simulink model "SecRwLtStArmScrnIsPosChk"  (R2018b)
settings: Solver=FixedStepDiscrete  StartTime=0.0  StopTime=10.0  FixedStep=0.01  RelTol=1e-3
undefined symbols (not defined in the file or in its folder): KeSMSuSecRwStArmTochPosDelta_Val, KeSMSuSecRwStArmTochPosTolr_Val
libraries: simulink x5, StIsPosChkLib x4
settings Model: Creator=sn2xws  LastModifiedBy=sn2xws
settings DataIOCC: SaveFormat=StructureWithTime
settings OptimizationCC: DefaultParameterBehavior=Inlined  EnhancedBackFolding=on  PassReuseOutputArgsAs=Individual arguments  ZeroExternalMemoryAtStartup=off  ZeroInternalMemoryAtStartup=off  OptimizeBlockOrder=speed  DifferentSizesBufferReuse=on  OptimizationCustomize=off
settings DebuggingCC: ParameterTunabilityLossMsg=error
settings ModelReferenceCC: ModelReferenceNumInstancesAllowed=Single
settings SFSimCC: MATLABDynamicMemAlloc=off
settings RTWCC: SystemTargetFile=autosar.tlc  GenCodeOnly=on  TemplateMakefile=ert_default_tmf  Description=AUTOSAR  GenerateReport=on  IncludeHyperlinkInReport=on  LaunchReport=on  GenerateTraceInfo=on  GenerateTraceReport=on  GenerateTraceReportSl=on  GenerateTraceReportSf=on  GenerateTraceReportEml=on  GenerateCodeMetricsReport=on
settings CodeAppCC: ForceParamTrailComments=on  IgnoreCustomStorageClasses=off  OperatorAnnotations=on  SimulinkDataObjDesc=on  SFDataObjDesc=on  InsertBlockDesc=on
settings STFCustomTargetCC: TargetLangStandard=C99 (ISO)  MultiwordLength=256  ParMdlRefBuildCompliant=on  CompOptLevelCompliant=on  IncludeMdlTerminateFcn=off  CombineOutputUpdateFcns=on  SuppressErrorStatus=on  ERTCustomFileBanners=on  SupportNonFinite=off  SupportComplex=off  SupportContinuousTime=off  SupportNonInlinedSFcns=off  RemoveResetFunc=on  MATLABClassNameForMDSCustomization=Simulink.SoftwareTarget.ERTCustomization  AutosarCompliant=on  UseToolchainInfoCompliant=on  LookupTableObjectStructAxisOrder=2,1,3,4,...  LUTObjectStructOrderEvenSpacing=Size,Table,Breakpoints  SystemTargetFile=autosar.tlc
settings ERTTargetCC: TargetLangStandard=C99 (ISO)  ConcurrentExecutionCompliant=off  IncludeMdlTerminateFcn=off  SuppressErrorStatus=on  SupportNonFinite=off  SupportComplex=off  ModelStepFunctionPrototypeControlCompliant=off  CPPClassGenCompliant=off  AutosarCompliant=on  LookupTableObjectStructAxisOrder=2,1,3,4,...  LUTObjectStructOrderEvenSpacing=Size,Table,Breakpoints  InlinedParameterPlacement=NonHierarchical  ERTCustomFileTemplate=example_file_process.tlc  ERTFilePackagingFormat=Compact

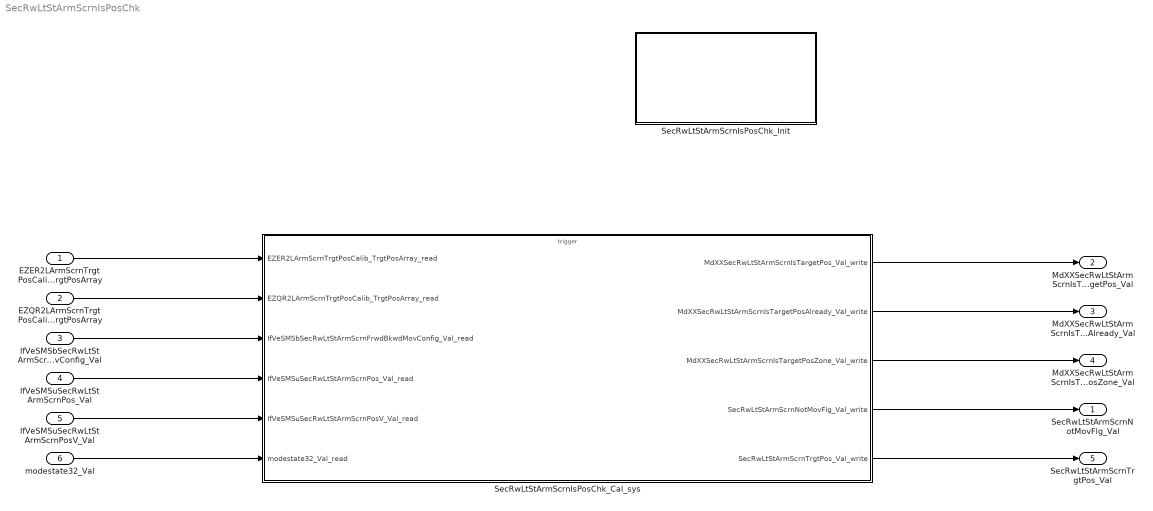
== system SecRwLtStArmScrnIsPosChk ==
  EZER2LArmScrnTrgtPosCalib_TrgtPosArray : Inport  Description=|  OutDataTypeStr=uint16  PortDimensions=3
      | 0:Pos
      | 1:Max
      | 2:Min
  EZQR2LArmScrnTrgtPosCalib_TrgtPosArray : Inport  Description=|  Port=2  OutDataTypeStr=uint16  PortDimensions=3
      | 0:Pos
      | 1:Max
      | 2:Min
  IfVeSMSbSecRwLtStArmScrnFrwdBkwdMovConfig_Val : Inport  Port=3  OutDataTypeStr=boolean  PortDimensions=1
  IfVeSMSuSecRwLtStArmScrnPos_Val : Inport  Port=4  OutDataTypeStr=uint16  PortDimensions=1
  IfVeSMSuSecRwLtStArmScrnPosV_Val : Inport  Port=5  OutDataTypeStr=boolean  PortDimensions=1
  modestate32_Val : Inport  Port=6  OutDataTypeStr=uint32  PortDimensions=1
  SecRwLtStArmScrnIsPosChk_Cal_sys : Subsystem
  SecRwLtStArmScrnIsPosChk_Init : Subsystem
  SecRwLtStArmScrnNotMovFlg_Val : Outport  OutDataTypeStr=boolean  PortDimensions=1
  MdXXSecRwLtStArmScrnIsTargetPos_Val : Outport  Port=2  OutDataTypeStr=uint32  PortDimensions=1
  MdXXSecRwLtStArmScrnIsTargetPosAlready_Val : Outport  Port=3  OutDataTypeStr=uint32  PortDimensions=1
  MdXXSecRwLtStArmScrnIsTargetPosZone_Val : Outport  Port=4  OutDataTypeStr=uint32  PortDimensions=1
  SecRwLtStArmScrnTrgtPos_Val : Outport  Port=5  OutDataTypeStr=uint16  PortDimensions=1
  wires:
  EZER2LArmScrnTrgtPosCalib_TrgtPosArray/1 -> SecRwLtStArmScrnIsPosChk_Cal_sys/1(EZER2LArmScrnTrgtPosCalib_TrgtPosArray_read)
  EZQR2LArmScrnTrgtPosCalib_TrgtPosArray/1 -> SecRwLtStArmScrnIsPosChk_Cal_sys/2(EZQR2LArmScrnTrgtPosCalib_TrgtPosArray_read)
  IfVeSMSbSecRwLtStArmScrnFrwdBkwdMovConfig_Val/1 -> SecRwLtStArmScrnIsPosChk_Cal_sys/3(IfVeSMSbSecRwLtStArmScrnFrwdBkwdMovConfig_Val_read)
  IfVeSMSuSecRwLtStArmScrnPos_Val/1 -> SecRwLtStArmScrnIsPosChk_Cal_sys/4(IfVeSMSuSecRwLtStArmScrnPos_Val_read)
  IfVeSMSuSecRwLtStArmScrnPosV_Val/1 -> SecRwLtStArmScrnIsPosChk_Cal_sys/5(IfVeSMSuSecRwLtStArmScrnPosV_Val_read)
  modestate32_Val/1 -> SecRwLtStArmScrnIsPosChk_Cal_sys/6(modestate32_Val_read)
  SecRwLtStArmScrnIsPosChk_Cal_sys/5(SecRwLtStArmScrnTrgtPos_Val_write) -> SecRwLtStArmScrnTrgtPos_Val/1
  SecRwLtStArmScrnIsPosChk_Cal_sys/1(MdXXSecRwLtStArmScrnIsTargetPos_Val_write) -> MdXXSecRwLtStArmScrnIsTargetPos_Val/1
  SecRwLtStArmScrnIsPosChk_Cal_sys/2(MdXXSecRwLtStArmScrnIsTargetPosAlready_Val_write) -> MdXXSecRwLtStArmScrnIsTargetPosAlready_Val/1
  SecRwLtStArmScrnIsPosChk_Cal_sys/3(MdXXSecRwLtStArmScrnIsTargetPosZone_Val_write) -> MdXXSecRwLtStArmScrnIsTargetPosZone_Val/1
  SecRwLtStArmScrnIsPosChk_Cal_sys/4(SecRwLtStArmScrnNotMovFlg_Val_write) -> SecRwLtStArmScrnNotMovFlg_Val/1

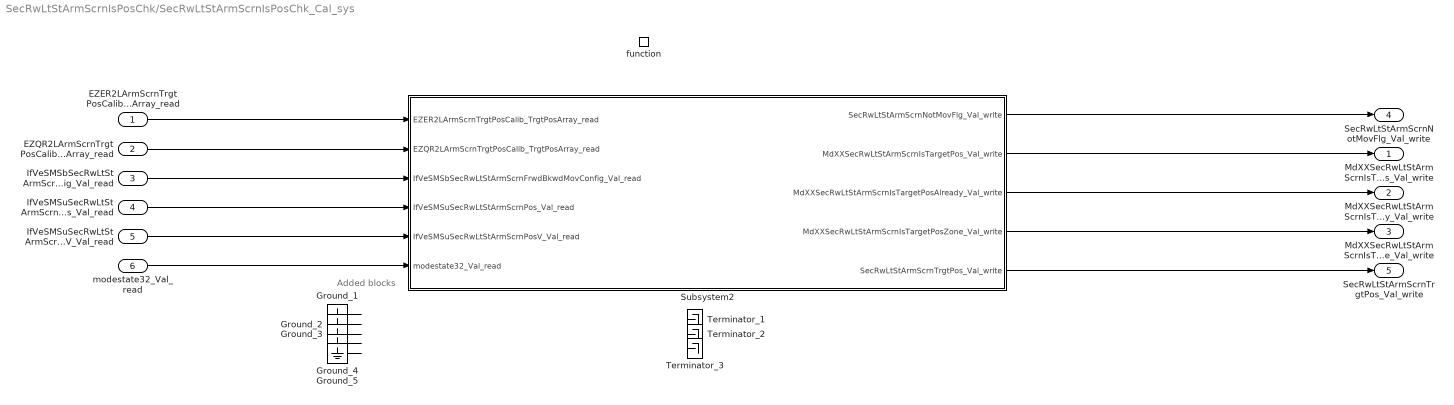
== system SecRwLtStArmScrnIsPosChk/SecRwLtStArmScrnIsPosChk_Cal_sys ==
  note: Added blocks
  EZER2LArmScrnTrgtPosCalib_TrgtPosArray_read : Inport
  EZQR2LArmScrnTrgtPosCalib_TrgtPosArray_read : Inport  Port=2
  IfVeSMSbSecRwLtStArmScrnFrwdBkwdMovConfig_Val_read : Inport  Port=3
  IfVeSMSuSecRwLtStArmScrnPos_Val_read : Inport  Port=4
  IfVeSMSuSecRwLtStArmScrnPosV_Val_read : Inport  Port=5
  modestate32_Val_read : Inport  Port=6
  function : TriggerPort  TriggerType=function-call  IsSimulinkFunction=on  FunctionName=SecRwLtStArmScrnIsPosChk_Cal  VariantControl=(inherit)
  Ground_{1..5} (5 alike) : Ground
  Subsystem2 : Subsystem
  Terminator_1 : Terminator
  Terminator_2 : Terminator
  Terminator_3 : Terminator
  MdXXSecRwLtStArmScrnIsTargetPos_Val_write : Outport
      settings: EnsureOutportIsVirtual=on
  MdXXSecRwLtStArmScrnIsTargetPosAlready_Val_write : Outport  Port=2
      settings: EnsureOutportIsVirtual=on
  MdXXSecRwLtStArmScrnIsTargetPosZone_Val_write : Outport  Port=3
      settings: EnsureOutportIsVirtual=on
  SecRwLtStArmScrnNotMovFlg_Val_write : Outport  Port=4
      settings: EnsureOutportIsVirtual=on
  SecRwLtStArmScrnTrgtPos_Val_write : Outport  Port=5
      settings: EnsureOutportIsVirtual=on
  wires:
  EZER2LArmScrnTrgtPosCalib_TrgtPosArray_read/1 -> Subsystem2/1(EZER2LArmScrnTrgtPosCalib_TrgtPosArray_read)
  EZQR2LArmScrnTrgtPosCalib_TrgtPosArray_read/1 -> Subsystem2/2(EZQR2LArmScrnTrgtPosCalib_TrgtPosArray_read)
  IfVeSMSbSecRwLtStArmScrnFrwdBkwdMovConfig_Val_read/1 -> Subsystem2/3(IfVeSMSbSecRwLtStArmScrnFrwdBkwdMovConfig_Val_read)
  IfVeSMSuSecRwLtStArmScrnPos_Val_read/1 -> Subsystem2/4(IfVeSMSuSecRwLtStArmScrnPos_Val_read)
  IfVeSMSuSecRwLtStArmScrnPosV_Val_read/1 -> Subsystem2/5(IfVeSMSuSecRwLtStArmScrnPosV_Val_read)
  modestate32_Val_read/1 -> Subsystem2/6(modestate32_Val_read)
  Subsystem2/1(SecRwLtStArmScrnNotMovFlg_Val_write) -> SecRwLtStArmScrnNotMovFlg_Val_write/1
  Subsystem2/2(MdXXSecRwLtStArmScrnIsTargetPos_Val_write) -> MdXXSecRwLtStArmScrnIsTargetPos_Val_write/1
  Subsystem2/3(MdXXSecRwLtStArmScrnIsTargetPosAlready_Val_write) -> MdXXSecRwLtStArmScrnIsTargetPosAlready_Val_write/1
  Subsystem2/4(MdXXSecRwLtStArmScrnIsTargetPosZone_Val_write) -> MdXXSecRwLtStArmScrnIsTargetPosZone_Val_write/1
  Subsystem2/5(SecRwLtStArmScrnTrgtPos_Val_write) -> SecRwLtStArmScrnTrgtPos_Val_write/1
  Ground_1/1 -> ?
  Ground_2/1 -> ?
  Ground_3/1 -> ?
  Ground_4/1 -> ?
  Ground_5/1 -> ?
  ? -> Terminator_1/1
  ? -> Terminator_2/1
  ? -> Terminator_3/1

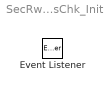
== system SecRwLtStArmScrnIsPosChk/SecRwLtStArmScrnIsPosChk_Init ==
  Event Listener : EventListener  EventName=reset

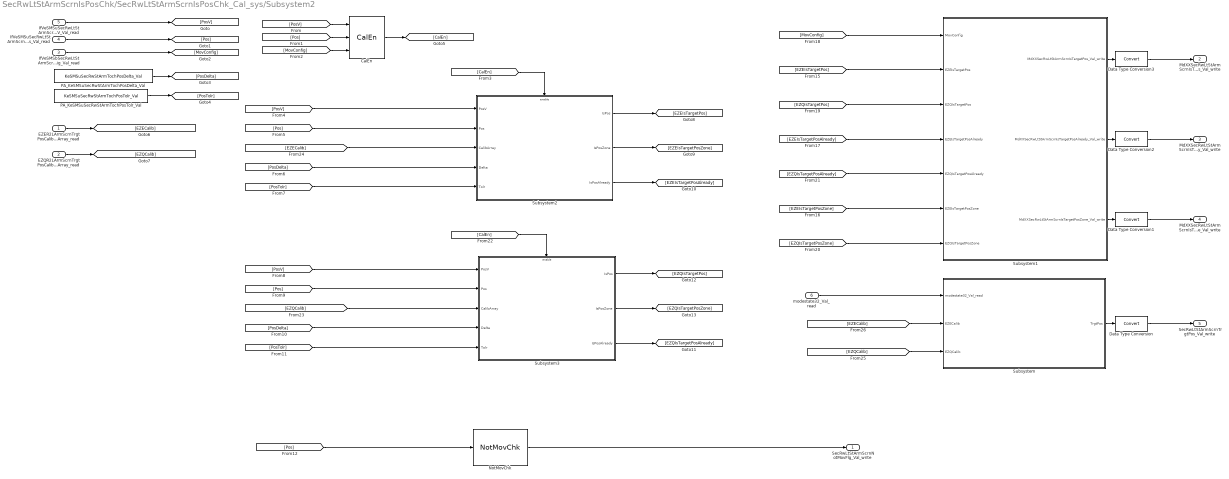
== system SecRwLtStArmScrnIsPosChk/SecRwLtStArmScrnIsPosChk_Cal_sys/Subsystem2 ==
  EZER2LArmScrnTrgtPosCalib_TrgtPosArray_read : Inport
  EZQR2LArmScrnTrgtPosCalib_TrgtPosArray_read : Inport  Port=2
  IfVeSMSbSecRwLtStArmScrnFrwdBkwdMovConfig_Val_read : Inport  Port=3
  IfVeSMSuSecRwLtStArmScrnPos_Val_read : Inport  Port=4
  IfVeSMSuSecRwLtStArmScrnPosV_Val_read : Inport  Port=5
  modestate32_Val_read : Inport  Port=6
  CalEn : StIsPosChkLib/CalEn  SystemSampleTime=-1
  Data Type Conversion{,1..3} (4 alike) : DataTypeConversion
  NotMovChk : StIsPosChkLib/NotMovChk  SystemSampleTime=-1
  PA_KeSMSuSecRwStArmTochPosDelta_Val : Constant  Value=KeSMSuSecRwStArmTochPosDelta_Val
  PA_KeSMSuSecRwStArmTochPosTolr_Val : Constant  Value=KeSMSuSecRwStArmTochPosTolr_Val
  Subsystem : Subsystem
  Subsystem1 : Subsystem
  Subsystem2 : Subsystem
  Subsystem3 : Subsystem
  SecRwLtStArmScrnNotMovFlg_Val_write : Outport
      settings: EnsureOutportIsVirtual=on
  MdXXSecRwLtStArmScrnIsTargetPos_Val_write : Outport  Port=2
      settings: EnsureOutportIsVirtual=on
  MdXXSecRwLtStArmScrnIsTargetPosAlready_Val_write : Outport  Port=3
      settings: EnsureOutportIsVirtual=on
  MdXXSecRwLtStArmScrnIsTargetPosZone_Val_write : Outport  Port=4
      settings: EnsureOutportIsVirtual=on
  SecRwLtStArmScrnTrgtPos_Val_write : Outport  Port=5
      settings: EnsureOutportIsVirtual=on
  wires:
  [PosV] -> Subsystem2/1(PosV)
  EZQR2LArmScrnTrgtPosCalib_TrgtPosArray_read/1 -> [EZQCalib]
  PA_KeSMSuSecRwStArmTochPosDelta_Val/1 -> [PosDelta]
  [MovConfig] -> Subsystem1/1(MovConfig)
  IfVeSMSuSecRwLtStArmScrnPosV_Val_read/1 -> [PosV]
  Subsystem3/1(IsPos) -> [EZQIsTargetPos]
  Data Type Conversion2/1 -> MdXXSecRwLtStArmScrnIsTargetPosAlready_Val_write/1
  NotMovChk/1 -> SecRwLtStArmScrnNotMovFlg_Val_write/1
  Data Type Conversion3/1 -> MdXXSecRwLtStArmScrnIsTargetPos_Val_write/1
  PA_KeSMSuSecRwStArmTochPosTolr_Val/1 -> [PosTolr]
  [EZEIsTargetPos] -> Subsystem1/2(EZEIsTargetPos)
  [PosDelta] -> Subsystem2/4(Delta)
  [PosDelta] -> Subsystem3/4(Delta)
  [PosTolr] -> Subsystem2/5(Tolr)
  [Pos] -> Subsystem2/2(Pos)
  Data Type Conversion/1 -> SecRwLtStArmScrnTrgtPos_Val_write/1
  Subsystem1/2(MdXXSecRwLtStArmScrnIsTargetPosAlready_Val_write) -> Data Type Conversion2/1
  [EZQIsTargetPos] -> Subsystem1/3(EZQIsTargetPos)
  Subsystem3/3(IsPosAlready) -> [EZQIsTargetPosAlready]
  Subsystem1/1(MdXXSecRwLtStArmScrnIsTargetPos_Val_write) -> Data Type Conversion3/1
  [Pos] -> NotMovChk/1
  Subsystem2/2(IsPosZone) -> [EZEIsTargetPosZone]
  [PosTolr] -> Subsystem3/5(Tolr)
  modestate32_Val_read/1 -> Subsystem/1(modestate32_Val_read)
  Subsystem2/1(IsPos) -> [EZEIsTargetPos]
  Subsystem/1(TrgtPos) -> Data Type Conversion/1
  [Pos] -> CalEn/2
  Subsystem2/3(IsPosAlready) -> [EZEIsTargetPosAlready]
  [PosV] -> Subsystem3/1(PosV)
  [EZQIsTargetPosAlready] -> Subsystem1/5(EZQIsTargetPosAlready)
  [EZQCalib] -> Subsystem3/3(CalibArray)
  [CalEn] -> Subsystem2/Enable
  [EZEIsTargetPosAlready] -> Subsystem1/4(EZEIsTargetPosAlready)
  IfVeSMSuSecRwLtStArmScrnPos_Val_read/1 -> [Pos]
  [CalEn] -> Subsystem3/Enable
  [PosV] -> CalEn/1
  [EZECalib] -> Subsystem2/3(CalibArray)
  [EZEIsTargetPosZone] -> Subsystem1/6(EZEIsTargetPosZone)
  Subsystem3/2(IsPosZone) -> [EZQIsTargetPosZone]
  [Pos] -> Subsystem3/2(Pos)
  [MovConfig] -> CalEn/3
  CalEn/1 -> [CalEn]
  [EZQCalib] -> Subsystem/3(EZQCalib)
  Subsystem1/3(MdXXSecRwLtStArmScrnIsTargetPosZone_Val_write) -> Data Type Conversion1/1
  Data Type Conversion1/1 -> MdXXSecRwLtStArmScrnIsTargetPosZone_Val_write/1
  [EZQIsTargetPosZone] -> Subsystem1/7(EZQIsTargetPosZone)
  EZER2LArmScrnTrgtPosCalib_TrgtPosArray_read/1 -> [EZECalib]
  IfVeSMSbSecRwLtStArmScrnFrwdBkwdMovConfig_Val_read/1 -> [MovConfig]
  [EZECalib] -> Subsystem/2(EZECalib)

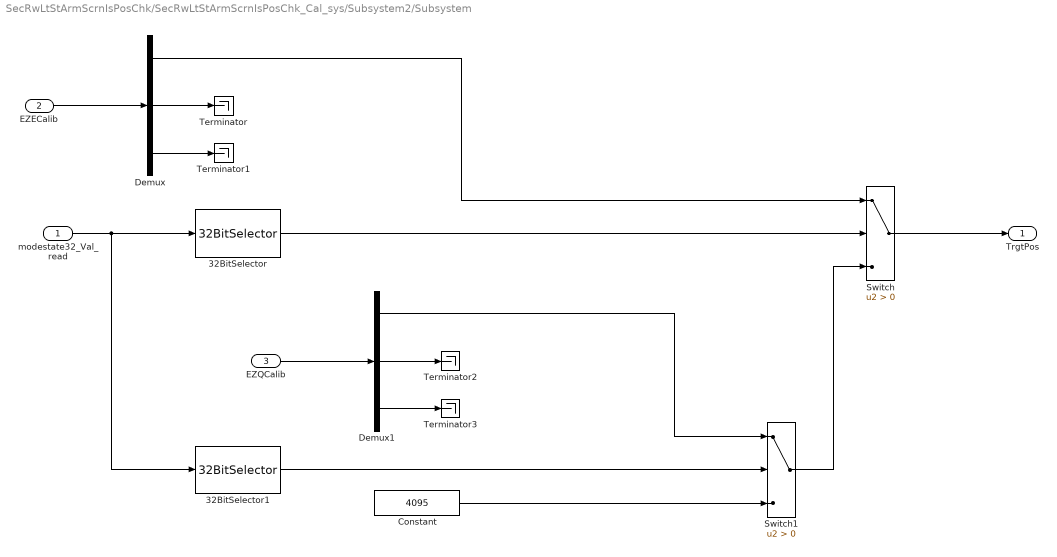
== system SecRwLtStArmScrnIsPosChk/SecRwLtStArmScrnIsPosChk_Cal_sys/Subsystem2/Subsystem ==
  modestate32_Val_read : Inport
  EZECalib : Inport  Port=2
  EZQCalib : Inport  Port=3
  32BitSelector : StIsPosChkLib/32BitSelector  BitNum=0
  32BitSelector1 : StIsPosChkLib/32BitSelector  BitNum=3
  Constant : Constant  Value=4095  OutDataTypeStr=uint16
  Demux : Demux  Outputs=3
  Demux1 : Demux  Outputs=3
  Switch : Switch  Criteria=u2 > Threshold
  Switch1 : Switch  Criteria=u2 > Threshold
  Terminator{,1..3} (4 alike) : Terminator
  TrgtPos : Outport
      settings: EnsureOutportIsVirtual=on
  wires:
  32BitSelector/1 -> Switch/2
  modestate32_Val_read/1 -> 32BitSelector1/1, 32BitSelector/1
  Demux/1 -> Switch/1
  Demux/3 -> Terminator1/1
  Demux/2 -> Terminator/1
  EZECalib/1 -> Demux/1
  EZQCalib/1 -> Demux1/1
  Demux1/2 -> Terminator2/1
  Demux1/3 -> Terminator3/1
  Demux1/1 -> Switch1/1
  Switch/1 -> TrgtPos/1
  Switch1/1 -> Switch/3
  32BitSelector1/1 -> Switch1/2
  Constant/1 -> Switch1/3

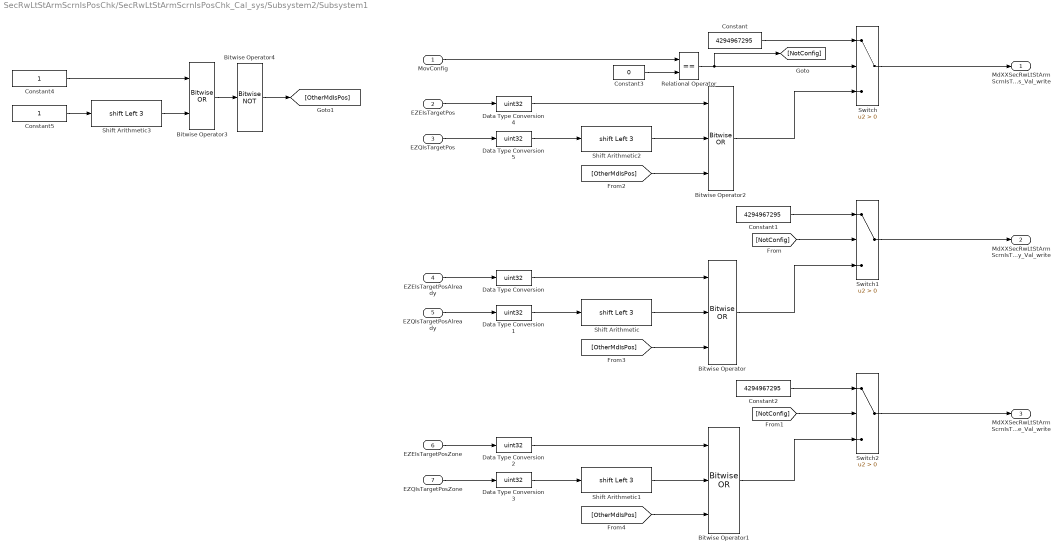
== system SecRwLtStArmScrnIsPosChk/SecRwLtStArmScrnIsPosChk_Cal_sys/Subsystem2/Subsystem1 ==
  MovConfig : Inport
  EZEIsTargetPos : Inport  Port=2
  EZQIsTargetPos : Inport  Port=3
  EZEIsTargetPosAlready : Inport  Port=4
  EZQIsTargetPosAlready : Inport  Port=5
  EZEIsTargetPosZone : Inport  Port=6
  EZQIsTargetPosZone : Inport  Port=7
  Bitwise Operator : simulink/Logic and Bit Operations/Bitwise Operator  logicop=OR  UseBitMask=off  NumInputPorts=3  BitMask=bin2dec('11011001')  BitMaskRealWorld=Stored Integer
  Bitwise Operator1 : simulink/Logic and Bit Operations/Bitwise Operator  logicop=OR  UseBitMask=off  NumInputPorts=3  BitMask=bin2dec('11011001')  BitMaskRealWorld=Stored Integer
  Bitwise Operator2 : simulink/Logic and Bit Operations/Bitwise Operator  logicop=OR  UseBitMask=off  NumInputPorts=3  BitMask=bin2dec('11011001')  BitMaskRealWorld=Stored Integer
  Bitwise Operator3 : simulink/Logic and Bit Operations/Bitwise Operator  logicop=OR  UseBitMask=off  NumInputPorts=2  BitMask=bin2dec('11011001')  BitMaskRealWorld=Stored Integer
  Bitwise Operator4 : simulink/Logic and Bit Operations/Bitwise Operator  logicop=NOT  UseBitMask=off  BitMask=bin2dec('11011001')  BitMaskRealWorld=Stored Integer
  Constant : Constant  Value=4294967295  OutDataTypeStr=uint32
  Constant1 : Constant  Value=4294967295  OutDataTypeStr=uint32
  Constant2 : Constant  Value=4294967295  OutDataTypeStr=uint32
  Constant3 : Constant  Value=0  OutDataTypeStr=uint8
  Constant4 : Constant  OutDataTypeStr=uint32
  Constant5 : Constant  OutDataTypeStr=uint32
  Data Type Conversion{,1..5} (6 alike) : DataTypeConversion  OutDataTypeStr=uint32
  Relational Operator : RelationalOperator  Operator===  OutDataTypeStr=boolean  RndMeth=Simplest
  Shift Arithmetic{,1..3} (4 alike) : ArithShift  BitShiftNumber=3  BitShiftDirection=Left
  Switch : Switch  Criteria=u2 > Threshold
  Switch1 : Switch  Criteria=u2 > Threshold
  Switch2 : Switch  Criteria=u2 > Threshold
  MdXXSecRwLtStArmScrnIsTargetPos_Val_write : Outport
      settings: EnsureOutportIsVirtual=on
  MdXXSecRwLtStArmScrnIsTargetPosAlready_Val_write : Outport  Port=2
      settings: EnsureOutportIsVirtual=on
  MdXXSecRwLtStArmScrnIsTargetPosZone_Val_write : Outport  Port=3
      settings: EnsureOutportIsVirtual=on
  wires:
  Constant3/1 -> Relational Operator/2
  Constant/1 -> Switch/1
  Relational Operator/1 -> [NotConfig], Switch/2
  MovConfig/1 -> Relational Operator/1
  Switch/1 -> MdXXSecRwLtStArmScrnIsTargetPos_Val_write/1
  [NotConfig] -> Switch1/2
  Constant1/1 -> Switch1/1
  Switch1/1 -> MdXXSecRwLtStArmScrnIsTargetPosAlready_Val_write/1
  Switch2/1 -> MdXXSecRwLtStArmScrnIsTargetPosZone_Val_write/1
  Constant2/1 -> Switch2/1
  [NotConfig] -> Switch2/2
  Data Type Conversion1/1 -> Shift Arithmetic/1
  Data Type Conversion/1 -> Bitwise Operator/1
  Shift Arithmetic/1 -> Bitwise Operator/2
  Shift Arithmetic1/1 -> Bitwise Operator1/2
  Data Type Conversion2/1 -> Bitwise Operator1/1
  Data Type Conversion3/1 -> Shift Arithmetic1/1
  Bitwise Operator1/1 -> Switch2/3
  Bitwise Operator/1 -> Switch1/3
  Shift Arithmetic2/1 -> Bitwise Operator2/2
  Data Type Conversion4/1 -> Bitwise Operator2/1
  Data Type Conversion5/1 -> Shift Arithmetic2/1
  Bitwise Operator2/1 -> Switch/3
  EZEIsTargetPos/1 -> Data Type Conversion4/1
  EZQIsTargetPos/1 -> Data Type Conversion5/1
  EZQIsTargetPosZone/1 -> Data Type Conversion3/1
  EZEIsTargetPosZone/1 -> Data Type Conversion2/1
  EZQIsTargetPosAlready/1 -> Data Type Conversion1/1
  EZEIsTargetPosAlready/1 -> Data Type Conversion/1
  Constant5/1 -> Shift Arithmetic3/1
  Shift Arithmetic3/1 -> Bitwise Operator3/2
  Constant4/1 -> Bitwise Operator3/1
  Bitwise Operator3/1 -> Bitwise Operator4/1
  Bitwise Operator4/1 -> [OtherMdIsPos]
  [OtherMdIsPos] -> Bitwise Operator2/3
  [OtherMdIsPos] -> Bitwise Operator/3
  [OtherMdIsPos] -> Bitwise Operator1/3

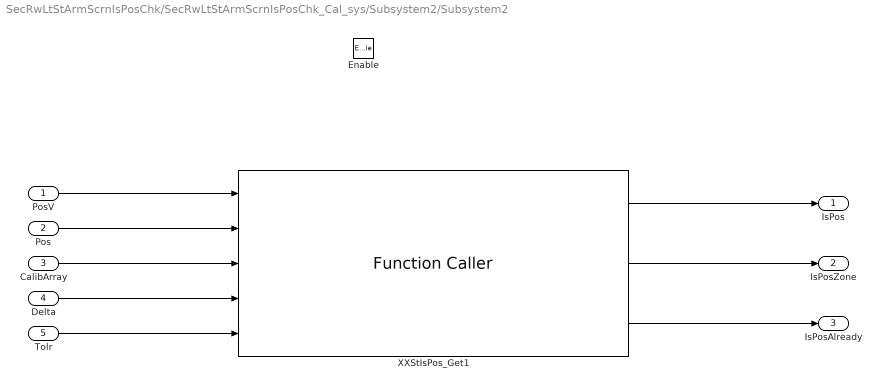
== system SecRwLtStArmScrnIsPosChk/SecRwLtStArmScrnIsPosChk_Cal_sys/Subsystem2/Subsystem2 ==
  PosV : Inport
  Pos : Inport  Port=2
  CalibArray : Inport  Port=3
  Delta : Inport  Port=4
  Tolr : Inport  Port=5
  Enable : EnablePort
  XXStIsPos_Get1 : FunctionCaller  FunctionPrototype=[IsPos,IsPosZone,IsPosAlready] = XXStIsPos_Get(PosV,Pos,CalibArray,Delta,Tolr)  InputArgumentSpecifications=boolean(true), uint16(1), uint16([1;1;1]), uint16(1), uint16(1)  OutputArgumentSpecifications=boolean(true), boolean(true), boolean(true)
  IsPos : Outport
  IsPosZone : Outport  Port=2
  IsPosAlready : Outport  Port=3
  wires:
  XXStIsPos_Get1/3 -> IsPosAlready/1
  Pos/1 -> XXStIsPos_Get1/2
  XXStIsPos_Get1/2 -> IsPosZone/1
  PosV/1 -> XXStIsPos_Get1/1
  CalibArray/1 -> XXStIsPos_Get1/3
  XXStIsPos_Get1/1 -> IsPos/1
  Delta/1 -> XXStIsPos_Get1/4
  Tolr/1 -> XXStIsPos_Get1/5

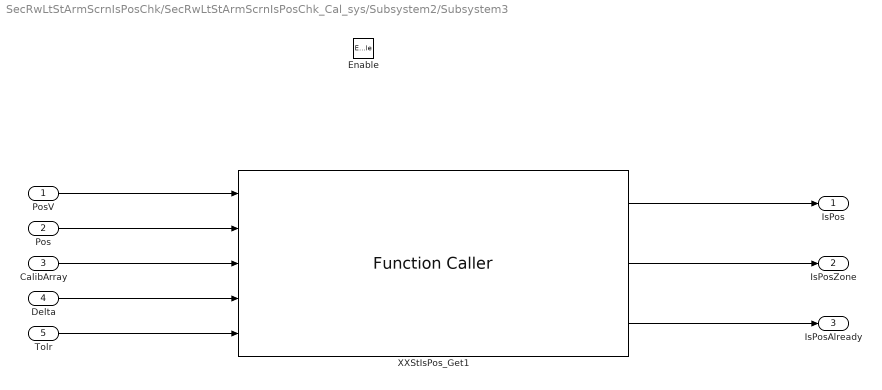
== system SecRwLtStArmScrnIsPosChk/SecRwLtStArmScrnIsPosChk_Cal_sys/Subsystem2/Subsystem3 ==
  PosV : Inport
  Pos : Inport  Port=2
  CalibArray : Inport  Port=3
  Delta : Inport  Port=4
  Tolr : Inport  Port=5
  Enable : EnablePort
  XXStIsPos_Get1 : FunctionCaller  FunctionPrototype=[IsPos,IsPosZone,IsPosAlready] = XXStIsPos_Get(PosV,Pos,CalibArray,Delta,Tolr)  InputArgumentSpecifications=boolean(true), uint16(1), uint16([1;1;1]), uint16(1), uint16(1)  OutputArgumentSpecifications=boolean(true), boolean(true), boolean(true)
  IsPos : Outport
  IsPosZone : Outport  Port=2
  IsPosAlready : Outport  Port=3
  wires:
  Tolr/1 -> XXStIsPos_Get1/5
  Delta/1 -> XXStIsPos_Get1/4
  XXStIsPos_Get1/1 -> IsPos/1
  CalibArray/1 -> XXStIsPos_Get1/3
  PosV/1 -> XXStIsPos_Get1/1
  XXStIsPos_Get1/2 -> IsPosZone/1
  Pos/1 -> XXStIsPos_Get1/2
  XXStIsPos_Get1/3 -> IsPosAlready/1
